simulink library "sfundemos"  (Simulink 7.6)
settings: Solver=ode45  SolverMode=SingleTasking  StartTime=0.0  StopTime=10.0  RelTol=1e-3
Description:
  | Custom Code and Hand Coded Blocks using the S-function API
  | 
  | This library launches examples of different types of Simulink(R) S-functions. Simulink
  | S-functions allow you to extend Simulink with new hand coded blocks, interface
  | to custom external code, and create live interfaces to other programs. Models
  | containing S-functions in the following programming languages can be accessed
  |  through this demonstration: C, C++, M and Fortran.
  | 
  | Each example contains a model that exercises an S-function block and a link for
  | editing the S-function code. You can also access the main S-function file by
  | using the Edit... button on the S-function block dialog (which is under a mask in
  | some of the models; use the "Look Under Mask" context menu item to access the
  | S-function dialog in this situation).
  | 
  | Additionally, the S-function Builder block is a masked version of the S-function
  | block that includes an easy to use editor that automatically builds an S-function
  | out of a core algorithm that you enter into it along with input, output, and parameter
  | attributes. By default, the S-function Builder also creates a TLC file for use with
  | Real-Time Workshop(R) and Real-Time Workshop(R) Embedded Coder(TM).
settings Model: Creator=The MathWorks Inc.  CovMetricSettings=d  ExtModeAutoUpdateStatusClock=off

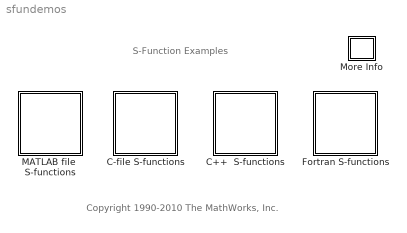
== system sfundemos ==
  note: S-Function Examples
  note: Copyright 1990-2010 The MathWorks, Inc.
  C++  S-functions : Subsystem
      mask Display: disp('C++')
  C-file S-functions : Subsystem
      mask Display: disp('C-files')
  Fortran S-functions : Subsystem
      mask Display: disp('Fortran')
  MATLAB file  S-functions : Subsystem
      mask Display: disp('MATLAB')
  More Info : Subsystem
      settings: OpenFcn=showdemo(bdroot(gcb))
      mask Display: disp('?')

== system sfundemos/C++  S-functions ==
  C++ Objects : Subsystem  mask{A=}
      mask prompts: A "Nedded to invoke correct OpenFcn from Browser:"
      settings: OpenFcn=sfundemo_open('sfcndemo_counter_cpp')
      mask Display: disp(sprintf('C++\nObjects'));
  Subsystem : Subsystem
      settings: OpenFcn=sfundemo_open('sfcndemo_cppcount')
      mask Display: disp(sprintf('C++ Simulink\nIntegration'));

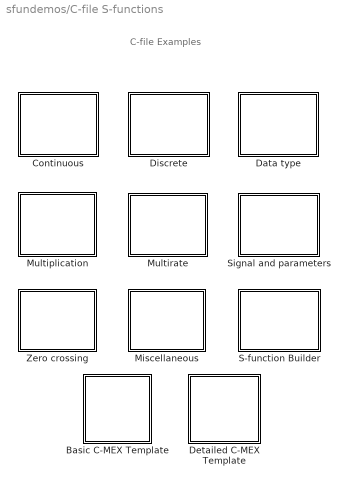
== system sfundemos/C-file S-functions ==
  note: C-file Examples
  "Basic C-MEX Template " : Subsystem  mask{a=}
      mask prompts: a "Needed to invoke correct OpenFcn in Browser"
      settings: OpenFcn=evalin('base','edit(fullfile(matlabroot,''simulink'',''src'',''sfuntmpl_basic.c''))')
      mask Display:
      | plot([.8  0 0 1 1 .8 .8 1],[1 1 0 0 .7 .7 1 .7])
      | disp('Basic\nC-MEX\nTemplate');
  Continuous : Subsystem
      mask Display: disp('Continuous')
  Data type : Subsystem
      mask Display: disp('Data type')
  Detailed C-MEX Template : Subsystem  mask{a=}
      mask prompts: a "Needed to invoke correct OpenFcn in Browser"
      settings: OpenFcn=evalin('base','edit(fullfile(matlabroot,''simulink'',''src'',''sfuntmpl_doc.c''))')
      mask Display:
      | plot([.8  0 0 1 1 .8 .8 1],[1 1 0 0 .7 .7 1 .7])
      | disp('Detailed\nC-MEX\nTemplate');
  Discrete : Subsystem
      mask Display: disp('Discrete')
  Miscellaneous : Subsystem
      mask Display: disp('Miscellaneous')
  Multiplication : Subsystem
      mask Display: disp('Multiplication')
  Multirate : Subsystem
      mask Display: disp('Multirate')
  S-function Builder : Subsystem
      mask Display: disp('S-function\nBuilder')
  Signal and parameters : Subsystem
      mask Display: disp('Signals and\nparameters')
  Zero crossing : Subsystem
      mask Display: disp('Zero crossing')

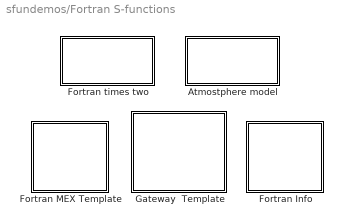
== system sfundemos/Fortran S-functions ==
  Atmostphere model : Subsystem  mask{A=}
      mask prompts: A "Needed to execute the correct OpenFcn from Browser:"
      settings: OpenFcn=sfundemo_open('sfcndemo_atmos')
      mask Display: disp('Atmosphere\nModel\nC calling Fortran');
  Fortran times two : Subsystem  mask{A=}
      mask prompts: A "Needed to execute the correct OpenFcn from Browser:"
      settings: OpenFcn=sfundemo_open('sfcndemo_timestwo_for')
      mask Display: disp('Times two\n(y=2*u)\nFortran');
  Fortran Info : Subsystem  mask{A=}
      mask prompts: A "Needed to invoke correct OpenFcn from Browser:"
      settings: OpenFcn=helpview([docroot, '/mapfiles/simulink.map'], 'creating_fortran_s-functions')
      mask Display:
      | plot([.8  0 0 1 1 .8 .8 1],[1 1 0 0 .7 .7 1 .7])
      | disp('Fortran\nMEX and\nC Gateway\nInfo');
  Fortran MEX Template : Subsystem  mask{A=}
      mask prompts: A "Needed to invoke correct OpenFcn from Browser:"
      settings: OpenFcn=evalin('base','edit(fullfile(matlabroot,''simulink'',''src'',''sfuntmpl_fortran.F''))')
      mask Display:
      | plot([.8  0 0 1 1 .8 .8 1],[1 1 0 0 .7 .7 1 .7])
      | disp('Fortran\nMEX\nTemplate');
  Gateway  Template : Subsystem  mask{A=}
      mask prompts: A "Needed to invoke correct OpenFcn from Browser:"
      settings: OpenFcn=evalin('base','edit(fullfile(matlabroot,''simulink'',''src'',''sfuntmpl_gate_fortran.c''))')
      mask Display:
      | plot([.8  0 0 1 1 .8 .8 1],[1 1 0 0 .7 .7 1 .7])
      | disp('C -> Fortran\nGateway\nTemplate');

== system sfundemos/MATLAB file  S-functions ==
  note: Note: Level 1 MATLAB file S-functions are provided to ensure
      | Simulink models with predecessor S-functions simulate properly.
      | Use Level-2 MATLAB file S-functions to develop new S-functions.
  Level-1 MATLAB file  S-functions : Subsystem
      mask Display: disp('Level-1 \nMATLAB files')
  Level-2  MATLAB file  S-functions : Subsystem
      mask Display: disp('Level-2 \nMATLAB files')

== system sfundemos/More Info ==

== system sfundemos/C++  S-functions/C++ Objects ==
  Gain : Gain  SaturateOnIntegerOverflow=on  OutDataTypeStr=Inherit: Same as input  ParamDataTypeStr=Inherit: Same as input

== system sfundemos/C++  S-functions/Subsystem ==
  Gain : Gain

== system sfundemos/C-file S-functions/Basic C-MEX Template  ==
  Gain : Gain  SaturateOnIntegerOverflow=on  OutDataTypeStr=Inherit: Same as input  ParamDataTypeStr=Inherit: Same as input

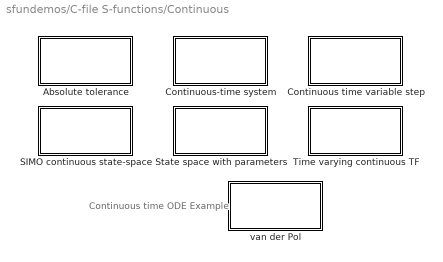
== system sfundemos/C-file S-functions/Continuous ==
  note: Continuous time
      | ODE
      | Example
  Absolute tolerance : Subsystem  mask{A=}
      mask prompts: A "Needed to execute the correct OpenFcn from Browser:"
      settings: OpenFcn=sfundemo_open('sfcndemo_sfun_atol')
      mask Display: disp('Absolute tolerance');
  Continuous time variable step : Subsystem  mask{A=}
      mask prompts: A "Needed to execute the correct OpenFcn from Browser:"
      settings: OpenFcn=sfundemo_open('sfcndemo_vsfunc')
      mask Display: disp('Continuous time\nvariable step');
  Continuous-time system : Subsystem  mask{Q=}
      mask prompts: Q "Needed to execute the correct OpenFcn from Browser:"
      settings: OpenFcn=sfundemo_open('sfcndemo_csfunc')
      mask Display: disp('Continuous time\nsystem');
  SIMO continuous state-space : Subsystem  mask{Q=}
      mask prompts: Q "Needed to execute the correct OpenFcn from Browser:"
      settings: OpenFcn=sfundemo_open('sfcndemo_simomex')
      mask Display: disp('SIMO continuous\nstate-space');
  State space with parameters : Subsystem  mask{A=}
      mask prompts: A "Needed to execute the correct OpenFcn from Browser:"
      settings: OpenFcn=sfundemo_open('sfcndemo_stspace')
      mask Display: disp('State space\nwith parameters');
  Time varying continuous TF : Subsystem  mask{Q=}
      mask prompts: Q "Needed to execute the correct OpenFcn from Browser:"
      settings: OpenFcn=sfundemo_open('sfcndemo_stvctf')
      mask Display: disp('Time varying\ncontinuous\ntransfer function');
  van der Pol : Subsystem  mask{A=}
      mask prompts: A "Needed to execute the correct OpenFcn from Browser:"
      settings: OpenFcn=sfundemo_open('sfcndemo_vdpmex')
      mask Display: disp(' van der Pol\nequation');

== system sfundemos/C-file S-functions/Data type ==
  Complex signal support : Subsystem  mask{a=}
      mask prompts: a "Needed to execute the correct OpenFcn from Browser:"
      settings: OpenFcn=sfundemo_open('sfcndemo_cplx')
      mask Display: disp('Complex signal \nsupport');
  Data typed parameters : Subsystem  mask{A=}
      mask prompts: A "Needed to execute the correct OpenFcn from Browser:"
      settings: OpenFcn=sfundemo_open('sfcndemo_dtype_param')
      mask Display: disp('Data typed\nParameters');
  Data typed I/O : Subsystem  mask{a=}
      mask prompts: a "Needed to execute the correct OpenFcn from Browser:"
      settings: OpenFcn=sfundemo_open('sfcndemo_dtype_io')
      mask Display: disp('Data typed\nI/O');

== system sfundemos/C-file S-functions/Detailed C-MEX Template ==
  Gain : Gain  SaturateOnIntegerOverflow=on  OutDataTypeStr=Inherit: Same as input  ParamDataTypeStr=Inherit: Same as input

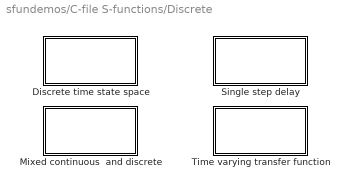
== system sfundemos/C-file S-functions/Discrete ==
  Discrete time state space : Subsystem  mask{A=}
      mask prompts: A "Needed to execute the correct OpenFcn from Browser:"
      settings: OpenFcn=sfundemo_open('sfcndemo_dsfunc')
      mask Display: disp('Discrete time\nstate space');
  Mixed continuous  and discrete : Subsystem  mask{A=}
      mask prompts: A "Needed to execute the correct OpenFcn from Browser:"
      settings: OpenFcn=sfundemo_open('sfcndemo_mixedmex')
      mask Display: disp('Mixed continuous\ndiscrete states');
  Single step delay : Subsystem  mask{A=}
      mask prompts: A "Needed to execute the correct OpenFcn from Browser:"
      settings: OpenFcn=sfundemo_open('sfcndemo_sfunmem')
      mask Display: disp('Memory\n(single step delay)');
  Time varying transfer function : Subsystem  mask{A=}
      mask prompts: A "Needed to execute the correct OpenFcn from Browser:"
      settings: OpenFcn=sfundemo_open('sfcndemo_stvdtf')
      mask Display: disp('Time varying\ndiscrete\ntransfer function');

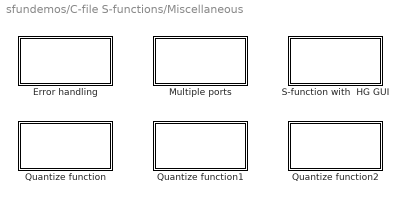
== system sfundemos/C-file S-functions/Miscellaneous ==
  Error handling : Subsystem  mask{a=}
      mask prompts: a "Needed to execute the correct OpenFcn from Browser:"
      settings: OpenFcn=sfundemo_open('sfcndemo_sfun_errhdl')
      mask Display: disp('Error\nhandling');
  Multiple ports : Subsystem  mask{a=}
      mask prompts: a "Needed to execute the correct OpenFcn from Browser:"
      settings: OpenFcn=sfundemo_open('sfcndemo_sfun_multiport')
      mask Display: disp('Multiple ports');
  Quantize function : Subsystem  mask{a=}
      mask prompts: a "Needed to execute the correct OpenFcn from Browser:"
      settings: OpenFcn=sfundemo_open('sfcndemo_sfun_quantize')
      mask Display: disp('Quantize\nfunction');
  Quantize function1 : Subsystem  mask{a=}
      mask prompts: a "Needed to execute the correct OpenFcn from Browser:"
      settings: OpenFcn=sfundemo_open('sfcndemo_sfun_rtwdwork')
      mask Display: disp('Dwork RTW\nproperties');
  Quantize function2 : Subsystem  mask{a=}
      mask prompts: a "Needed to execute the correct OpenFcn from Browser:"
      settings: OpenFcn=sfundemo_open('sfcndemo_sfun_simstate')
      mask Display: disp('Simulation State');
  S-function with  HG GUI : Subsystem  mask{a=}
      mask prompts: a "Needed to execute the correct OpenFcn from Browser:"
      settings: OpenFcn=sfundemo_open('sfcndemo_hg_gui')
      mask Display: disp('S-function\nwith HG GUI');

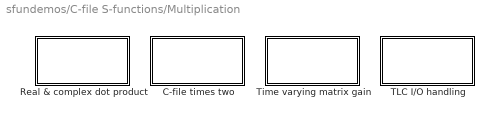
== system sfundemos/C-file S-functions/Multiplication ==
  C-file times two : Subsystem  mask{A=}
      mask prompts: A "Needed to execute the correct OpenFcn from Browser:"
      settings: OpenFcn=sfundemo_open('sfcndemo_timestwo')
      mask Display: disp('Times two\n(y=2*u)');
  Real & complex dot product : Subsystem  mask{A=}
      mask prompts: A "Needed to execute the correct OpenFcn from Browser:"
      settings: OpenFcn=sfundemo_open('sfcndemo_sdotproduct')
      mask Display: disp('Real & complex\ndot product');
  TLC I/O handling : Subsystem  mask{A=}
      mask prompts: A "Needed to execute the correct OpenFcn from Browser:"
      settings: OpenFcn=sfundemo_open('sfcndemo_io_handling')
      mask Display: disp(' TLC I/O\nHandling');
  Time varying matrix gain : Subsystem  mask{a=}
      mask prompts: a "Needed to execute the correct OpenFcn from Browser:"
      settings: OpenFcn=sfundemo_open('sfcndemo_stvmgain')
      mask Display: disp('Time varying\nmatrix gain');

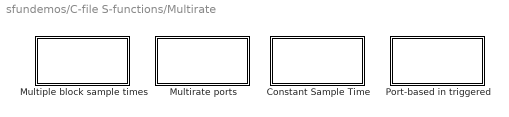
== system sfundemos/C-file S-functions/Multirate ==
  Constant Sample Time : Subsystem  mask{a=}
      mask prompts: a "Needed to execute the correct OpenFcn from Browser:"
      settings: OpenFcn=sfundemo_open('sfcndemo_port_constant')
      mask Display: disp('Constant sample\ntime on ports');
  Multiple block sample times : Subsystem  mask{a=}
      mask prompts: a "Needed to execute the correct OpenFcn from Browser:"
      settings: OpenFcn=sfundemo_open('sfcndemo_mixedm')
      mask Display: disp('Multiple\nblock sample times');
  Multirate ports : Subsystem  mask{a=}
      mask prompts: a "Needed to execute the correct OpenFcn from Browser:"
      settings: OpenFcn=sfundemo_open('sfcndemo_sfun_multirate')
      mask Display: disp('Multirate ports');
  Port-based in triggered : Subsystem  mask{a=}
      mask prompts: a "Needed to execute the correct OpenFcn from Browser:"
      settings: OpenFcn=sfundemo_open('sfcndemo_port_triggered')
      mask Display: disp('Port-based in\ntriggered');

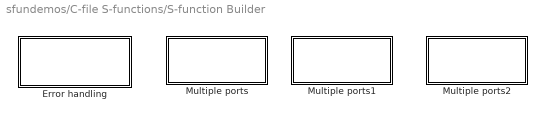
== system sfundemos/C-file S-functions/S-function Builder ==
  Error handling : Subsystem  mask{a=}
      mask prompts: a "Needed to execute the correct OpenFcn from Browser:"
      settings: AttributesFormatString=\n\n  OpenFcn=sfundemo_open('sfbuilder_euler2dc')
      mask Display: disp('Direct Cosine Matrix\nfrom Euler Angles ');
  Multiple ports : Subsystem  mask{a=}
      mask prompts: a "Needed to execute the correct OpenFcn from Browser:"
      settings: AttributesFormatString=\n\n  OpenFcn=sfundemo_open('sfbuilder_multiport')
      mask Display: disp('S-Function Builder\nwith multiple ports');
  Multiple ports1 : Subsystem  mask{a=}
      mask prompts: a "Needed to execute the correct OpenFcn from Browser:"
      settings: AttributesFormatString=\n\n  OpenFcn=sfundemo_open('sfbuilder_stats')
      mask Display: disp('Mean and Variance');
  Multiple ports2 : Subsystem  mask{a=}
      mask prompts: a "Needed to execute the correct OpenFcn from Browser:"
      settings: OpenFcn=sfundemo_open('sfbuilder_bususage')
      mask Display: disp('S-Function Builder\nwith buses');

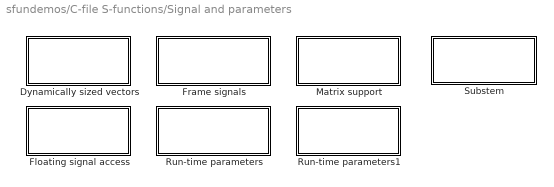
== system sfundemos/C-file S-functions/Signal and parameters ==
  Dynamically sized vectors : Subsystem  mask{a=}
      mask prompts: a "Needed to execute the correct OpenFcn from Browser:"
      settings: OpenFcn=sfundemo_open('sfcndemo_sfun_dynsize')
      mask Display: disp('Dynamically Sized\nVectors');
  Floating signal access : Subsystem  mask{a=}
      mask prompts: a "Needed to execute the correct OpenFcn from Browser:"
      settings: OpenFcn=sfundemo_open('sfcndemo_barplot')
      mask Display: disp('Floating Signal\nAccess\n(Bar Plot)');
  Frame signals : Subsystem  mask{a=}
      mask prompts: a "Needed to execute the correct OpenFcn from Browser:"
      settings: OpenFcn=sfundemo_open('sfcndemo_frame')
      mask Display: disp(sprintf('Frame Signals\n(Requires Signal\nProcessing Blockset)'));
  Matrix support : Subsystem  mask{a=}
      mask prompts: a "Needed to execute the correct OpenFcn from Browser:"
      settings: OpenFcn=sfundemo_open('sfcndemo_matadd')
      mask Display: disp('Matrix support');
  Run-time parameters : Subsystem  mask{s=}
      mask prompts: s "Needed to execute the correct OpenFcn from Browser:"
      settings: OpenFcn=sfundemo_open('sfcndemo_runtime')
      mask Display: disp('Run-time\nParameters');
  Run-time parameters1 : Subsystem  mask{s=}
      mask prompts: s "Needed to execute the correct OpenFcn from Browser:"
      settings: OpenFcn=sfundemo_open('sfcndemo_csparam')
      mask Display: disp('Context-sensitive\nParameters');
  Substem : Subsystem
      settings: OpenFcn=sfundemo_open('sfcndemo_varsize')
      mask Display: disp('Variable-Size\nSignals')

== system sfundemos/C-file S-functions/Zero crossing ==
  Zero crossing : Subsystem  mask{a=}
      mask prompts: a "Needed to execute the correct OpenFcn from Browser:"
      settings: OpenFcn=sfundemo_open('sfcndemo_sfun_zc')
      mask Display: disp('Zero\ncrossing');
  Zero crossing with saturation : Subsystem  mask{a=}
      mask prompts: a "Needed to execute the correct OpenFcn from Browser:"
      settings: OpenFcn=sfundemo_open('sfcndemo_sfun_zc_sat')
      mask Display: disp('Zero crossing\nwith saturation');

== system sfundemos/Fortran S-functions/Atmostphere model ==
  Gain : Gain  SaturateOnIntegerOverflow=on  OutDataTypeStr=Inherit: Same as input  ParamDataTypeStr=Inherit: Same as input

== system sfundemos/Fortran S-functions/Fortran times two ==
  Gain : Gain  SaturateOnIntegerOverflow=on  OutDataTypeStr=Inherit: Same as input  ParamDataTypeStr=Inherit: Same as input

== system sfundemos/Fortran S-functions/Fortran Info ==
  Gain : Gain  SaturateOnIntegerOverflow=on  OutDataTypeStr=Inherit: Same as input  ParamDataTypeStr=Inherit: Same as input

== system sfundemos/Fortran S-functions/Fortran MEX Template ==
  Gain : Gain  SaturateOnIntegerOverflow=on  OutDataTypeStr=Inherit: Same as input  ParamDataTypeStr=Inherit: Same as input

== system sfundemos/Fortran S-functions/Gateway  Template ==
  Gain : Gain  SaturateOnIntegerOverflow=on  OutDataTypeStr=Inherit: Same as input  ParamDataTypeStr=Inherit: Same as input

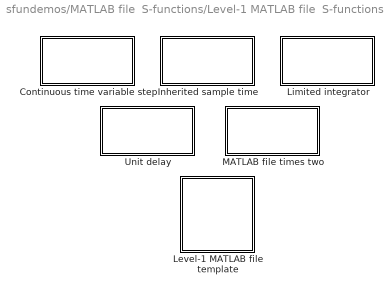
== system sfundemos/MATLAB file  S-functions/Level-1 MATLAB file  S-functions ==
  Continuous time variable step : Subsystem  mask{A=}
      mask prompts: A "Needed to invoke OpenFcn from the browser:"
      settings: OpenFcn=sfundemo_open('sfcndemo_vsfunc')
      mask Display: disp('Continuous time\nvariable step\nMATLAB file');
  Inherited sample time : Subsystem  mask{A=}
      mask prompts: A "Needed to invoke OpenFcn from the browser:"
      settings: OpenFcn=sfundemo_open('sfcndemo_sfundsc1')
      mask Display: disp('Inherited\nsample time');
  Level-1 MATLAB file template : Subsystem  mask{a=}
      mask prompts: a "Needed to invoke correct OpenFcn in Browser:"
      settings: OpenFcn=edit('sfuntmpl.m');
      mask Display:
      | plot([.8  0 0 1 1 .8 .8 1],[1 1 0 0 .7 .7 1 .7])
      | disp('Level-1 \nMATLAB file\nS-function\nTemplate')
  Limited integrator : Subsystem  mask{A=}
      mask prompts: A "Needed to invoke OpenFcn from the browser:"
      settings: OpenFcn=sfundemo_open('sfcndemo_limintm')
      mask Display: disp('Limited\nintegrator');
  MATLAB file times two : Subsystem  mask{A=}
      mask prompts: A "Needed to invoke OpenFcn from the browser:"
      settings: OpenFcn=sfundemo_open('sfcndemo_timestwo')
      mask Display: disp('Times two\n(y=2*u)\nMATLAB file');
  Unit delay : Subsystem  mask{A=}
      mask prompts: A "Needed to invoke OpenFcn from the browser:"
      settings: OpenFcn=sfundemo_open('sfcndemo_sfundsc2')
      mask Display: disp('Unit delay');

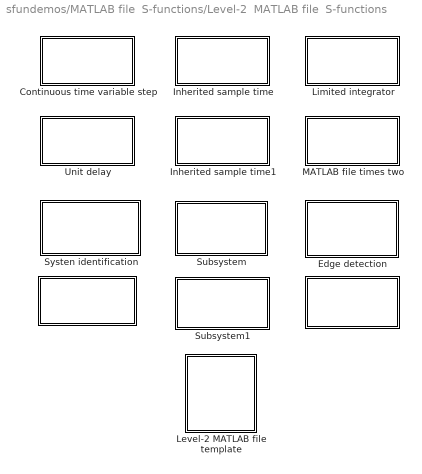
== system sfundemos/MATLAB file  S-functions/Level-2  MATLAB file  S-functions ==
  " " : Subsystem  mask{A=0}
      mask prompts: A "Needed to invoke OpenFcn from the browser:"
      settings: OpenFcn=sfundemo_open('msfcndemo_multirate')
      mask Display: disp('Multirate \nM S-function');
  "    " : Subsystem  mask{A=0}
      mask prompts: A "Needed to invoke OpenFcn from the browser:"
      settings: OpenFcn=sfundemo_open('msfcndemo_fi')
      mask Display: disp('Fixed-Point \nMultiplication');
  Continuous time variable step : Subsystem  mask{A=}
      mask prompts: A "Needed to invoke OpenFcn from the browser:"
      settings: OpenFcn=sfundemo_open('msfcndemo_vsfunc')
      mask Display: disp('Continuous time\nvariable step\nMATLAB file');
  Edge detection : Subsystem  mask{A=}
      mask prompts: A "Needed to invoke OpenFcn from the browser:"
      settings: OpenFcn=sfundemo_open('sldemo_msfcn_edge_detect')
      mask Display: disp('Image \nedge detection \nusing Sobel filter');
  Inherited sample time : Subsystem  mask{A=}
      mask prompts: A "Needed to invoke OpenFcn from the browser:"
      settings: OpenFcn=sfundemo_open('msfcndemo_sfundsc1')
      mask Display: disp('Inherited\nsample time');
  Inherited sample time1 : Subsystem  mask{A=}
      mask prompts: A "Needed to invoke OpenFcn from the browser:"
      settings: OpenFcn=sfundemo_open('msfcndemo_varpulse')
      mask Display: disp('Variable\npulse generator');
  Level-2 MATLAB file template : Subsystem  mask{a=}
      mask prompts: a "Needed to invoke correct OpenFcn in Browser:"
      settings: OpenFcn=edit('msfuntmpl.m');
      mask Display:
      | plot([.8  0 0 1 1 .8 .8 1],[1 1 0 0 .7 .7 1 .7])
      | disp('Level-2 \nMATLAB file\nS-function\nTemplate')
  Limited integrator : Subsystem  mask{A=}
      mask prompts: A "Needed to invoke OpenFcn from the browser:"
      settings: OpenFcn=sfundemo_open('msfcndemo_limintm')
      mask Display: disp('Limited\nintegrator');
  MATLAB file times two : Subsystem  mask{A=}
      mask prompts: A "Needed to invoke OpenFcn from the browser:"
      settings: OpenFcn=sfundemo_open('msfcndemo_timestwo')
      mask Display: disp('Times two\n(y=2*u)\nMATLAB file');
  Subsystem : Subsystem
      settings: OpenFcn=sfundemo_open('msfcndemo_varsize')
      mask Display: disp('Variable-Size\nSignals')
  Subsystem1 : Subsystem
      settings: OpenFcn=sfundemo_open('sldemo_msfcn_frame')
      mask Display: disp('Frame signals')
  Systen identification : Subsystem  mask{A=}
      mask prompts: A "Needed to invoke OpenFcn from the browser:"
      settings: OpenFcn=sfundemo_open('sldemo_msfcn_lms')
      mask Display: disp('System \n identification \n using LMS\n');
  Unit delay : Subsystem  mask{A=}
      mask prompts: A "Needed to invoke OpenFcn from the browser:"
      settings: OpenFcn=sfundemo_open('msfcndemo_sfundsc2')
      mask Display: disp('Unit delay');

== system sfundemos/C-file S-functions/Continuous/Absolute tolerance ==
  Gain : Gain  SaturateOnIntegerOverflow=on  OutDataTypeStr=Inherit: Same as input  ParamDataTypeStr=Inherit: Same as input

== system sfundemos/C-file S-functions/Continuous/Continuous time variable step ==
  Gain : Gain  SaturateOnIntegerOverflow=on  OutDataTypeStr=Inherit: Same as input  ParamDataTypeStr=Inherit: Same as input

== system sfundemos/C-file S-functions/Continuous/Continuous-time system ==
  Gain : Gain  SaturateOnIntegerOverflow=on  OutDataTypeStr=Inherit: Same as input  ParamDataTypeStr=Inherit: Same as input

== system sfundemos/C-file S-functions/Continuous/SIMO continuous state-space ==
  Gain : Gain  SaturateOnIntegerOverflow=on  OutDataTypeStr=Inherit: Same as input  ParamDataTypeStr=Inherit: Same as input

== system sfundemos/C-file S-functions/Continuous/State space with parameters ==
  Gain : Gain  SaturateOnIntegerOverflow=on  OutDataTypeStr=Inherit: Same as input  ParamDataTypeStr=Inherit: Same as input

== system sfundemos/C-file S-functions/Continuous/Time varying continuous TF ==
  Gain : Gain  SaturateOnIntegerOverflow=on  OutDataTypeStr=Inherit: Same as input  ParamDataTypeStr=Inherit: Same as input

== system sfundemos/C-file S-functions/Continuous/van der Pol ==
  Gain : Gain  SaturateOnIntegerOverflow=on  OutDataTypeStr=Inherit: Same as input  ParamDataTypeStr=Inherit: Same as input

== system sfundemos/C-file S-functions/Data type/Complex signal support ==
  Gain : Gain  SaturateOnIntegerOverflow=on  OutDataTypeStr=Inherit: Same as input  ParamDataTypeStr=Inherit: Same as input

== system sfundemos/C-file S-functions/Data type/Data typed parameters ==
  Gain : Gain  SaturateOnIntegerOverflow=on  OutDataTypeStr=Inherit: Same as input  ParamDataTypeStr=Inherit: Same as input

== system sfundemos/C-file S-functions/Data type/Data typed I/O ==
  Gain : Gain  SaturateOnIntegerOverflow=on  OutDataTypeStr=Inherit: Same as input  ParamDataTypeStr=Inherit: Same as input

== system sfundemos/C-file S-functions/Discrete/Discrete time state space ==
  Gain : Gain  SaturateOnIntegerOverflow=on  OutDataTypeStr=Inherit: Same as input  ParamDataTypeStr=Inherit: Same as input

== system sfundemos/C-file S-functions/Discrete/Mixed continuous  and discrete ==
  Gain : Gain  SaturateOnIntegerOverflow=on  OutDataTypeStr=Inherit: Same as input  ParamDataTypeStr=Inherit: Same as input

== system sfundemos/C-file S-functions/Discrete/Single step delay ==
  Gain : Gain  SaturateOnIntegerOverflow=on  OutDataTypeStr=Inherit: Same as input  ParamDataTypeStr=Inherit: Same as input

== system sfundemos/C-file S-functions/Discrete/Time varying transfer function ==
  Gain : Gain  SaturateOnIntegerOverflow=on  OutDataTypeStr=Inherit: Same as input  ParamDataTypeStr=Inherit: Same as input

== system sfundemos/C-file S-functions/Miscellaneous/Error handling ==
  Gain : Gain  SaturateOnIntegerOverflow=on  OutDataTypeStr=Inherit: Same as input  ParamDataTypeStr=Inherit: Same as input

== system sfundemos/C-file S-functions/Miscellaneous/Multiple ports ==
  Gain : Gain  SaturateOnIntegerOverflow=on  OutDataTypeStr=Inherit: Same as input  ParamDataTypeStr=Inherit: Same as input

== system sfundemos/C-file S-functions/Miscellaneous/Quantize function ==
  Gain : Gain  SaturateOnIntegerOverflow=on  OutDataTypeStr=Inherit: Same as input  ParamDataTypeStr=Inherit: Same as input

== system sfundemos/C-file S-functions/Miscellaneous/Quantize function1 ==
  Gain : Gain  SaturateOnIntegerOverflow=on  OutDataTypeStr=Inherit: Same as input  ParamDataTypeStr=Inherit: Same as input

== system sfundemos/C-file S-functions/Miscellaneous/Quantize function2 ==
  Gain : Gain  SaturateOnIntegerOverflow=on  OutDataTypeStr=Inherit: Same as input  ParamDataTypeStr=Inherit: Same as input

== system sfundemos/C-file S-functions/Miscellaneous/S-function with  HG GUI ==
  Gain : Gain  SaturateOnIntegerOverflow=on  OutDataTypeStr=Inherit: Same as input  ParamDataTypeStr=Inherit: Same as input

== system sfundemos/C-file S-functions/Multiplication/C-file times two ==
  Gain : Gain  SaturateOnIntegerOverflow=on  OutDataTypeStr=Inherit: Same as input  ParamDataTypeStr=Inherit: Same as input

== system sfundemos/C-file S-functions/Multiplication/Real & complex dot product ==
  Gain : Gain  SaturateOnIntegerOverflow=on  OutDataTypeStr=Inherit: Same as input  ParamDataTypeStr=Inherit: Same as input

== system sfundemos/C-file S-functions/Multiplication/TLC I/O handling ==
  Gain : Gain  SaturateOnIntegerOverflow=on  OutDataTypeStr=Inherit: Same as input  ParamDataTypeStr=Inherit: Same as input

== system sfundemos/C-file S-functions/Multiplication/Time varying matrix gain ==
  Gain : Gain  SaturateOnIntegerOverflow=on  OutDataTypeStr=Inherit: Same as input  ParamDataTypeStr=Inherit: Same as input

== system sfundemos/C-file S-functions/Multirate/Constant Sample Time ==
  Gain : Gain  SaturateOnIntegerOverflow=on  OutDataTypeStr=Inherit: Same as input  ParamDataTypeStr=Inherit: Same as input

== system sfundemos/C-file S-functions/Multirate/Multiple block sample times ==
  Gain : Gain  SaturateOnIntegerOverflow=on  OutDataTypeStr=Inherit: Same as input  ParamDataTypeStr=Inherit: Same as input

== system sfundemos/C-file S-functions/Multirate/Multirate ports ==
  Gain : Gain  SaturateOnIntegerOverflow=on  OutDataTypeStr=Inherit: Same as input  ParamDataTypeStr=Inherit: Same as input

== system sfundemos/C-file S-functions/Multirate/Port-based in triggered ==
  Gain : Gain  SaturateOnIntegerOverflow=on  OutDataTypeStr=Inherit: Same as input  ParamDataTypeStr=Inherit: Same as input

== system sfundemos/C-file S-functions/S-function Builder/Error handling ==
  Gain : Gain  SaturateOnIntegerOverflow=on  OutDataTypeStr=Inherit: Same as input  ParamDataTypeStr=Inherit: Same as input

== system sfundemos/C-file S-functions/S-function Builder/Multiple ports ==
  Gain : Gain  SaturateOnIntegerOverflow=on  OutDataTypeStr=Inherit: Same as input  ParamDataTypeStr=Inherit: Same as input

== system sfundemos/C-file S-functions/S-function Builder/Multiple ports1 ==
  Gain : Gain  SaturateOnIntegerOverflow=on  OutDataTypeStr=Inherit: Same as input  ParamDataTypeStr=Inherit: Same as input

== system sfundemos/C-file S-functions/S-function Builder/Multiple ports2 ==
  Gain : Gain  SaturateOnIntegerOverflow=on  OutDataTypeStr=Inherit: Same as input  ParamDataTypeStr=Inherit: Same as input

== system sfundemos/C-file S-functions/Signal and parameters/Dynamically sized vectors ==

== system sfundemos/C-file S-functions/Signal and parameters/Floating signal access ==

== system sfundemos/C-file S-functions/Signal and parameters/Frame signals ==

== system sfundemos/C-file S-functions/Signal and parameters/Matrix support ==

== system sfundemos/C-file S-functions/Signal and parameters/Run-time parameters ==

== system sfundemos/C-file S-functions/Signal and parameters/Run-time parameters1 ==

== system sfundemos/C-file S-functions/Signal and parameters/Substem ==
  Gain : Gain
  wires:
  ? -> Gain/1
  Gain/1 -> ?

== system sfundemos/C-file S-functions/Zero crossing/Zero crossing ==
  Gain : Gain  SaturateOnIntegerOverflow=on  OutDataTypeStr=Inherit: Same as input  ParamDataTypeStr=Inherit: Same as input

== system sfundemos/C-file S-functions/Zero crossing/Zero crossing with saturation ==
  Gain : Gain  SaturateOnIntegerOverflow=on  OutDataTypeStr=Inherit: Same as input  ParamDataTypeStr=Inherit: Same as input

== system sfundemos/MATLAB file  S-functions/Level-1 MATLAB file  S-functions/Continuous time variable step ==
  Gain : Gain  SaturateOnIntegerOverflow=on  OutDataTypeStr=Inherit: Same as input  ParamDataTypeStr=Inherit: Same as input

== system sfundemos/MATLAB file  S-functions/Level-1 MATLAB file  S-functions/Inherited sample time ==
  Gain : Gain  SaturateOnIntegerOverflow=on  OutDataTypeStr=Inherit: Same as input  ParamDataTypeStr=Inherit: Same as input

== system sfundemos/MATLAB file  S-functions/Level-1 MATLAB file  S-functions/Level-1 MATLAB file template ==
  SubSystem : Subsystem

== system sfundemos/MATLAB file  S-functions/Level-1 MATLAB file  S-functions/Limited integrator ==
  Gain : Gain  SaturateOnIntegerOverflow=on  OutDataTypeStr=Inherit: Same as input  ParamDataTypeStr=Inherit: Same as input

== system sfundemos/MATLAB file  S-functions/Level-1 MATLAB file  S-functions/MATLAB file times two ==
  Gain : Gain  SaturateOnIntegerOverflow=on  OutDataTypeStr=Inherit: Same as input  ParamDataTypeStr=Inherit: Same as input

== system sfundemos/MATLAB file  S-functions/Level-1 MATLAB file  S-functions/Unit delay ==
  Gain : Gain  SaturateOnIntegerOverflow=on  OutDataTypeStr=Inherit: Same as input  ParamDataTypeStr=Inherit: Same as input

== system sfundemos/MATLAB file  S-functions/Level-2  MATLAB file  S-functions/  ==

== system sfundemos/MATLAB file  S-functions/Level-2  MATLAB file  S-functions/     ==

== system sfundemos/MATLAB file  S-functions/Level-2  MATLAB file  S-functions/Continuous time variable step ==
  Gain : Gain  SaturateOnIntegerOverflow=on  OutDataTypeStr=Inherit: Same as input  ParamDataTypeStr=Inherit: Same as input

== system sfundemos/MATLAB file  S-functions/Level-2  MATLAB file  S-functions/Edge detection ==
  Gain : Gain  SaturateOnIntegerOverflow=on  OutDataTypeStr=Inherit: Same as input  ParamDataTypeStr=Inherit: Same as input

== system sfundemos/MATLAB file  S-functions/Level-2  MATLAB file  S-functions/Inherited sample time ==
  Gain : Gain  SaturateOnIntegerOverflow=on  OutDataTypeStr=Inherit: Same as input  ParamDataTypeStr=Inherit: Same as input

== system sfundemos/MATLAB file  S-functions/Level-2  MATLAB file  S-functions/Inherited sample time1 ==
  Gain : Gain  SaturateOnIntegerOverflow=on  OutDataTypeStr=Inherit: Same as input  ParamDataTypeStr=Inherit: Same as input

== system sfundemos/MATLAB file  S-functions/Level-2  MATLAB file  S-functions/Level-2 MATLAB file template ==
  SubSystem : Subsystem

== system sfundemos/MATLAB file  S-functions/Level-2  MATLAB file  S-functions/Limited integrator ==
  Gain : Gain  SaturateOnIntegerOverflow=on  OutDataTypeStr=Inherit: Same as input  ParamDataTypeStr=Inherit: Same as input

== system sfundemos/MATLAB file  S-functions/Level-2  MATLAB file  S-functions/MATLAB file times two ==
  Gain : Gain  SaturateOnIntegerOverflow=on  OutDataTypeStr=Inherit: Same as input  ParamDataTypeStr=Inherit: Same as input

== system sfundemos/MATLAB file  S-functions/Level-2  MATLAB file  S-functions/Subsystem ==
  Subsystem : Subsystem
  wires:
  ? -> Subsystem/1(In1)
  Subsystem/1(Out1) -> ?

== system sfundemos/MATLAB file  S-functions/Level-2  MATLAB file  S-functions/Subsystem1 ==
  Gain : Gain
  wires:
  ? -> Gain/1
  Gain/1 -> ?

== system sfundemos/MATLAB file  S-functions/Level-2  MATLAB file  S-functions/Systen identification ==
  Gain : Gain  SaturateOnIntegerOverflow=on  OutDataTypeStr=Inherit: Same as input  ParamDataTypeStr=Inherit: Same as input

== system sfundemos/MATLAB file  S-functions/Level-2  MATLAB file  S-functions/Unit delay ==
  Gain : Gain  SaturateOnIntegerOverflow=on  OutDataTypeStr=Inherit: Same as input  ParamDataTypeStr=Inherit: Same as input

== system sfundemos/MATLAB file  S-functions/Level-1 MATLAB file  S-functions/Level-1 MATLAB file template/SubSystem ==

== system sfundemos/MATLAB file  S-functions/Level-2  MATLAB file  S-functions/Level-2 MATLAB file template/SubSystem ==

== system sfundemos/MATLAB file  S-functions/Level-2  MATLAB file  S-functions/Subsystem/Subsystem ==
  In1 : Inport
  Gain : Gain
  Out1 : Outport
  wires:
  In1/1 -> Gain/1
  Gain/1 -> Out1/1
